simulink model "AdecuacionEMG4"  (Simulink 6.6)
settings: Solver=ode45  StartTime=0.0  StopTime=100  RelTol=1e-3
libraries: dsparch4 x2, dspwin32 x2, dspsnks4 x2, dspbuff3 x1, dspspect3 x1, dspstat3 x1
settings Model: Creator=F565la07hrfjn  LastModifiedBy=F565la07hrfjn
settings DebuggingCC: SolverPrmCheckMsg=none

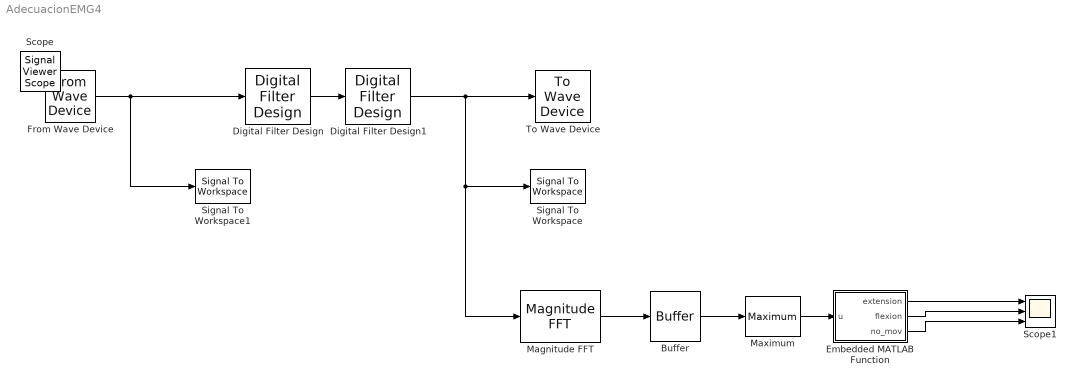
== system AdecuacionEMG4 ==
  Buffer : dspbuff3/Buffer  N=128  V=0  ic=0
  Digital Filter Design : dsparch4/Digital Filter Design  SystemSampleTime=-1  mwdsp_browser_bugfix_var=off
  Digital Filter Design1 : dsparch4/Digital Filter Design  SystemSampleTime=-1  mwdsp_browser_bugfix_var=off
  Embedded MATLAB Function : Stateflow chart
  From Wave Device : dspwin32/From Wave Device  SampleRate=44100  UserRate=16000  SampleWidth=8  Stereo=off  SamplesPerFrame=512  QueueDuration=3  useDefaultDevice=on  userDeviceID=Micrófono (Conexant High Defini  dType=double
  Magnitude FFT : dspspect3/Magnitude FFT  SystemSampleTime=-1  mag_or_magsq=Magnitude squared  fftLenInherit=off  fftsize=256
  Maximum : dspstat3/Maximum  DialogController=dspfixptddg.MinMax  DialogControllerArgs=DataTag2  fcn=Value  reset=None  indexBase=One  operateOver=Entire input  colComp=on  operation=maximum  roundingMode=Floor  overflowMode=off
  Scope1 : Scope  NumInputPorts=3
      settings: TimeRange=100  YMin=-1.5~-1.5~-1.5  YMax=1.5~1.5~1.5
  Signal To Workspace : dspsnks4/Signal To Workspace  SystemSampleTime=-1  VariableName=AF  FrameMode=Concatenate frames (2-D array)
      settings: FixptAsFi=off
  Signal To Workspace1 : dspsnks4/Signal To Workspace  SystemSampleTime=-1  VariableName=BF  FrameMode=Concatenate frames (2-D array)
      settings: FixptAsFi=off
  To Wave Device : dspwin32/To Wave Device  bufDuration=2  determineBufSize=on  userIntBufSize=256  initDelay=0.1  useDefaultDevice=on  userDeviceID=Altavoz y auricular interno (Co  enable24Bit=off
  Scope : SignalViewerScope  IOType=viewer  RefreshTime=0.035000
  wires:
  Digital Filter Design/1 -> Digital Filter Design1/1
  From Wave Device/1 -> Digital Filter Design/1, Signal To Workspace1/1
  Digital Filter Design1/1 -> Signal To Workspace/1, Magnitude FFT/1, To Wave Device/1
  Magnitude FFT/1 -> Buffer/1
  Buffer/1 -> Maximum/1
  Maximum/1 -> Embedded MATLAB Function/1(u)
  Embedded MATLAB Function/1(extension) -> Scope1/1
  Embedded MATLAB Function/2(flexion) -> Scope1/2
  Embedded MATLAB Function/3(no_mov) -> Scope1/3

== matlab function Embedded MATLAB Function ==
  data: u input inherited; extension output inherited; flexion output inherited; no_mov output inherited
function [extension,flexion,no_mov] = fcn(u)
% This block supports an embeddable subset of the MATLAB language.
% See the help menu for details. 

flexion=0;
no_mov=0;
extension=0;

if(u<100)
    flexion=0;
    no_mov=1;
    extension=0;
elseif(u>100&&u<2000)
    flexion=1;
    no_mov=0;
    extension=0;
elseif(u>2000)
    flexion=0;
    no_mov=0;
    extension=1;
end
